simulink model "UAV"  (R2018b)
settings: Solver=FixedStepAuto  StartTime=0.0  StopTime=10.0  RelTol=1e-3  EnableMultiTasking=on
values from neighbouring files (symbols this model uses):
  actuatorCentres = 0.0    [data.sldd]
  datcom : value not decoded    [data.sldd]
  deflectionLimits = -10.0    [data.sldd]
  envConsts = -1.3    [data.sldd]
  vehicle = 5.0    [data.sldd]
undefined symbols (not defined in the file or in its folder): aeroCoeff, Discrete, Time
libraries: simulink x28, ctrlSharedLib x8, arduinolib x7, aerolibasang x6, aerolibactuator x4, aerolibadyn x2, sharedTrackingLibrary x2, aerolibnav x2, shared6dof x1, aerolibanim x1, aerolibatmos2 x1, dspstat3 x1
(part 1 of 3)
settings Model: DataDictionary=data.sldd  VariantConfigurationObject=Sim_Mode  SimulationMode=accelerator  ExtModeTrigDuration=2  Creator=Aliak  LastModifiedBy=Aliak
settings OptimizationCC: DefaultUnderspecifiedDataType=single  EnhancedBackFolding=on  PassReuseOutputArgsAs=Individual arguments  LifeSpan=1  MaxStackSize=64  OptimizeBlockOrder=speed  DifferentSizesBufferReuse=on
settings DebuggingCC: ParameterTunabilityLossMsg=error
settings HardwareCC: ProdBitPerInt=16  ProdBitPerPointer=16  ProdBitPerSizeT=16  ProdBitPerPtrDiffT=16  ProdLargestAtomicFloat=None  ProdWordSize=8  ProdHWDeviceType=Atmel->AVR
settings SFSimCC: MATLABDynamicMemAlloc=off
settings RTWCC: SystemTargetFile=ert.tlc  HardwareBoard=Arduino Uno  TemplateMakefile=ert_default_tmf  GenerateReport=on  Toolchain=Arduino AVR  BuildConfiguration=Faster Runs  IncludeHyperlinkInReport=on  LaunchReport=on  GenerateTraceInfo=on  GenerateTraceReport=on  GenerateTraceReportSl=on  GenerateTraceReportSf=on  GenerateTraceReportEml=on  CheckMdlBeforeBuild=Warning
settings CodeAppCC: ForceParamTrailComments=on  IgnoreCustomStorageClasses=off  OperatorAnnotations=on  SimulinkDataObjDesc=on  SFDataObjDesc=on  InsertBlockDesc=on
settings ERTTargetCC: SupportContinuousTime=on  SupportVariableSizeSignals=on  CastingMode=Standards

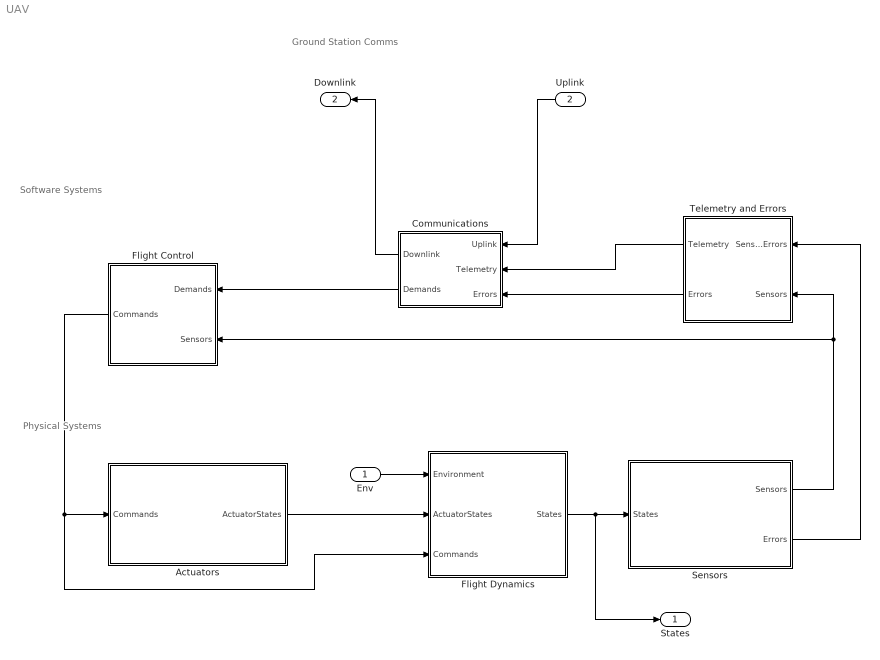
== system UAV ==
  note: Physical Systems
  note: Software Systems
  note: Ground Station Comms
  Env : Inport
  Uplink : Inport  Port=2  OutDataTypeStr=Bus: Uplink
  Actuators : Subsystem  Variant=on
  Communications : Subsystem
  Flight Control : Subsystem
  Flight Dynamics : Subsystem
  Sensors : Subsystem
  Telemetry and Errors : Subsystem  VariantControl=Variant1
  States : Outport  OutDataTypeStr=Bus: States
  Downlink : Outport  Port=2
  wires:
  Flight Dynamics/1(States) -> States/1, Sensors/1(States)
  Sensors/1(Sensors) -> Telemetry and Errors/2(Sensors), Flight Control/2(Sensors)
  Flight Control/1(Commands) -> Actuators/1(Commands), Flight Dynamics/3(Commands)
  Actuators/1(ActuatorStates) -> Flight Dynamics/2(ActuatorStates)
  Env/1 -> Flight Dynamics/1(Environment)
  Communications/2(Demands) -> Flight Control/1(Demands)
  Uplink/1 -> Communications/1(Uplink)
  Communications/1(Downlink) -> Downlink/1
  Sensors/2(Errors) -> Telemetry and Errors/1(SensorErrors)
  Telemetry and Errors/1(Telemetry) -> Communications/2(Telemetry)
  Telemetry and Errors/2(Errors) -> Communications/3(Errors)

== system UAV/Actuators ==
  Commands : Inport
  Model Actuators : Subsystem  VariantControl=SimType == 0
  Real Actuators : Subsystem  VariantControl=SimType == 2
  ActuatorStates : Outport

== system UAV/Communications ==
  Uplink : Inport  OutDataTypeStr=Bus: Uplink
  Telemetry : Inport  Port=2  OutDataTypeStr=Bus: Sensors
  Errors : Inport  Port=3  OutDataTypeStr=Bus: Errors
  Bus Creator : BusCreator  Inputs=6  OutDataTypeStr=Bus: Demands
      settings: InheritFromInputs=off
  Bus Selector : BusSelector  OutputSignals=AutoflightRefValues,ControlOverride
  Bus Selector1 : BusSelector  OutputSignals=FlightMode,HoldAltitude,HoldSpeed,HoldHeading,LLATarget
  Downlink : Outport
  Demands : Outport  Port=2  OutDataTypeStr=Bus: Demands
  wires:
  Uplink/1 -> Bus Selector/1
  Bus Selector/1 -> Bus Selector1/1  "<AutoflightRefValues>"
  Bus Selector1/1 -> Bus Creator/1  "<FlightMode>"
  Bus Selector1/2 -> Bus Creator/2  "<HoldAltitude>"
  Bus Selector1/3 -> Bus Creator/3  "<HoldSpeed>"
  Bus Selector1/4 -> Bus Creator/4  "<HoldHeading>"
  Bus Selector1/5 -> Bus Creator/5  "<LLATarget>"
  Bus Creator/1 -> Demands/1
  Bus Selector/2 -> Bus Creator/6  "<ControlOverride>"

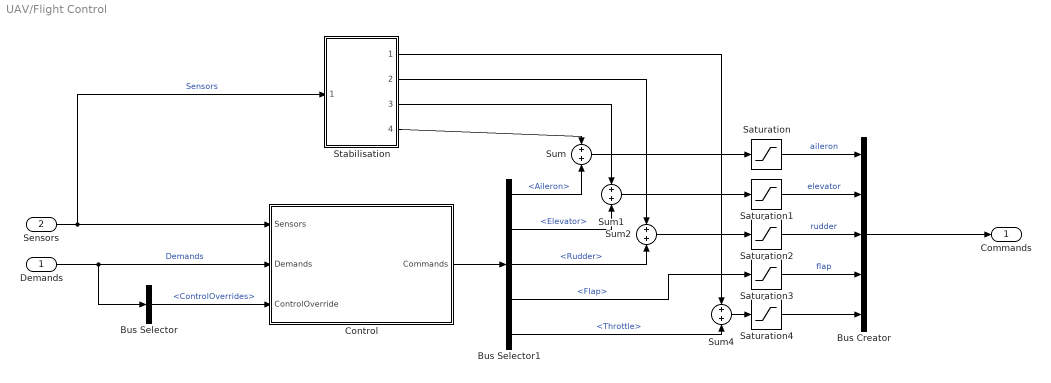
== system UAV/Flight Control ==
  Demands : Inport  OutDataTypeStr=Bus: Demands
  Sensors : Inport  Port=2  OutDataTypeStr=Bus: Sensors
  Bus Creator : BusCreator  Inputs=5  OutDataTypeStr=Bus: Commands
  Bus Selector : BusSelector  OutputSignals=ControlOverrides
  Bus Selector1 : BusSelector  OutputSignals=Aileron,Elevator,Rudder,Flap,Throttle
  Control : Stateflow chart  TreatAsAtomicUnit=on
  Saturation : Saturate  UpperLimit=deflectionLimits.aileron.max  LowerLimit=deflectionLimits.aileron.min
  Saturation1 : Saturate  UpperLimit=deflectionLimits.elevator.max  LowerLimit=deflectionLimits.elevator.min
  Saturation2 : Saturate  UpperLimit=deflectionLimits.rudder.max  LowerLimit=deflectionLimits.rudder.min
  Saturation3 : Saturate  UpperLimit=deflectionLimits.flap.max  LowerLimit=deflectionLimits.flap.min
  Saturation4 : Saturate  UpperLimit=1  LowerLimit=0
  Stabilisation : Subsystem
  Sum{,1..2,4} (4 alike) : Sum
  Commands : Outport
  wires:
  Bus Creator/1 -> Commands/1
  Sum/1 -> Saturation/1
  Sum1/1 -> Saturation1/1
  Sum2/1 -> Saturation2/1
  Saturation/1 -> Bus Creator/1  "aileron"
  Saturation1/1 -> Bus Creator/2  "elevator"
  Saturation2/1 -> Bus Creator/3  "rudder"
  Saturation3/1 -> Bus Creator/4  "flap"
  Control/1(Commands) -> Bus Selector1/1
  Bus Selector1/1 -> Sum/2  "<Aileron>"
  Sensors/1 -> Stabilisation/1(Sensors), Control/1(Sensors)  "Sensors"
  Demands/1 -> Bus Selector/1, Control/2(Demands)  "Demands"
  Bus Selector/1 -> Control/3(ControlOverride)  "<ControlOverrides>"
  Bus Selector1/2 -> Sum1/2  "<Elevator>"
  Bus Selector1/3 -> Sum2/2  "<Rudder>"
  Bus Selector1/4 -> Saturation3/1  "<Flap>"
  Sum4/1 -> Saturation4/1
  Bus Selector1/5 -> Sum4/2  "<Throttle>"
  Saturation4/1 -> Bus Creator/5
  Stabilisation/4(Roll Stab) -> Sum/1
  Stabilisation/3(Pitch Stab) -> Sum1/1
  Stabilisation/2(Yaw Stab) -> Sum2/1
  Stabilisation/1(Stall Stab) -> Sum4/1

== system UAV/Flight Dynamics ==
  Environment : Inport
  ActuatorStates : Inport  Port=2
  Commands : Inport  Port=3  OutDataTypeStr=Bus: Commands
  6DOF EOM : Subsystem  VariantControl=eom3DOF
  Bus Selector : BusSelector  OutputSignals=throttle
  Coeff Model : Subsystem  Commented=on  VariantControl=AeroModel==2
  DATCOM Model : Subsystem  VariantControl=AeroModel==1
  Propulsion : Subsystem
      settings: RTWSystemCode=Inline
  Sum1 : Sum  Inputs=|++  SaturateOnIntegerOverflow=on  InputSameDT=on  OutDataTypeStr=Inherit: Same as first input
  Sum2 : Sum  Inputs=|++  SaturateOnIntegerOverflow=on  InputSameDT=on  OutDataTypeStr=Inherit: Same as first input
  Visualization : Subsystem
  States : Outport  OutDataTypeStr=Bus: States
  wires:
  Commands/1 -> Bus Selector/1
  Sum2/1 -> 6DOF EOM/2(Forces)
  6DOF EOM/1(States) -> DATCOM Model/2(States), States/1, Visualization/1(States)
  Propulsion/1(F) -> Sum2/2
  Propulsion/2(M) -> Sum1/2
  Sum1/1 -> 6DOF EOM/3(Moments)
  Environment/1 -> DATCOM Model/1(Env), 6DOF EOM/1(Env)
  Bus Selector/1 -> Propulsion/1(cmd)  "<throttle>"
  ActuatorStates/1 -> DATCOM Model/3(ActuatorStates)
  DATCOM Model/1(F) -> Sum2/1
  DATCOM Model/2(M) -> Sum1/1

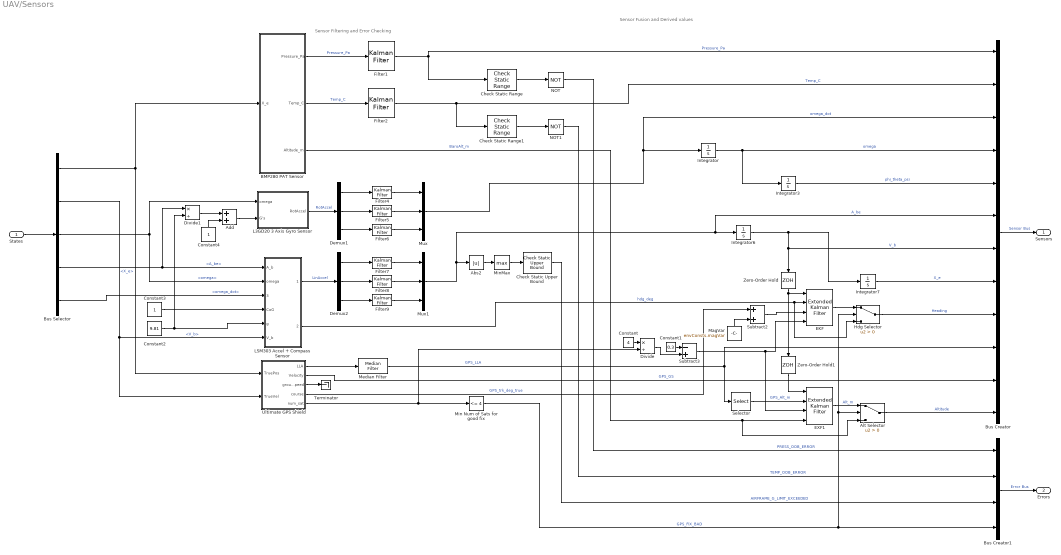
== system UAV/Sensors ==
  note: Sensor Fusion and Derived values
  note: Sensor Filtering and Error Checking
  States : Inport  OutDataTypeStr=Bus: States
  Abs2 : Abs
  Add : Sum
  Alt Selector : Switch  Criteria=u2 > Threshold  OutDataTypeStr=single  SaturateOnIntegerOverflow=on  InputSameDT=on
  "BMP280 PAT Sensor " : Subsystem
  Bus Creator : BusCreator  Inputs=12  OutDataTypeStr=Bus: Sensors
  Bus Creator1 : BusCreator  Inputs=4  OutDataTypeStr=Bus: Errors
  Bus Selector : BusSelector  OutputSignals=X_e,V_b,omega,A_be,omega_dot
  Check Static Range : simulink/Model Verification/Check  Static Range  Description=97025 <= u <= 104325  max=104325  max_included=on  min=97025  min_included=on  enabled=off  stopWhenAssertionFail=off  export=on  icon=graphic
      settings: SourceProductName=Simulink  SourceProductBaseCode=SL
  Check Static Range1 : simulink/Model Verification/Check  Static Range  Description=-10 <= u <= 30  max=30  max_included=on  min=-10  min_included=on  enabled=off  stopWhenAssertionFail=off  export=on  icon=graphic
      settings: SourceProductName=Simulink  SourceProductBaseCode=SL
  Check Static Upper Bound : simulink/Model Verification/Check Static  Upper Bound  Description=u <= 5  max=5  max_included=on  enabled=off  stopWhenAssertionFail=off  export=on  icon=graphic
      settings: SourceProductName=Simulink  SourceProductBaseCode=SL
  Constant : Constant  Value=4
  Constant1 : Constant  Value=0.3
  Constant2 : Constant  Value=9.81
  Constant3 : Constant
  Constant4 : Constant
  Demux1 : Demux  Outputs=3
  Demux2 : Demux  Outputs=3
  Divide : Product  Inputs=*/  OutMin=0.5  OutMax=30  OutDataTypeStr=Inherit: Inherit via back propagation  SaturateOnIntegerOverflow=on
  Divide1 : Product  Inputs=*/
  EKF : sharedTrackingLibrary/Extended Kalman Filter  StateTransitionFcn=headingStateTransitionFunc  HasStateTransitionJacobianFcn=off  HasAdditiveProcessNoise=Additive  ProcessNoise=1  HasTimeVaryingProcessNoise=off  HasStateTransitionFcnExtraArgument=1  InitialState=0  InitialStateCovariance=3  MeasurementFcn1=baroMeasurementFunc  HasMeasurementJacobianFcn1=off  HasMeasurementEnablePort1=off  HasAdditiveMeasurementNoise1=Additive  MeasurementNoise1=0.5  HasTimeVaryingMeasurementNoise1=off  HasMeasurementFcnExtraArgument1=0  MeasurementFcn2=gpsMeasurementFunc  HasMeasurementJacobianFcn2=off  HasMeasurementEnablePort2=off  HasAdditiveMeasurementNoise2=Additive  MeasurementNoise2=1  HasTimeVaryingMeasurementNoise2=on  HasMeasurementFcnExtraArgument2=0  MeasurementFcn3=myMeasurementFcn  HasMeasurementJacobianFcn3=off  HasMeasurementEnablePort3=off  HasAdditiveMeasurementNoise3=Additive  MeasurementNoise3=1  HasTimeVaryingMeasurementNoise3=off  HasMeasurementFcnExtraArgument3=0  MeasurementFcn4=myMeasurementFcn  HasMeasurementJacobianFcn4=off  HasMeasurementEnablePort4=off  HasAdditiveMeasurementNoise4=Additive  MeasurementNoise4=1  HasTimeVaryingMeasurementNoise4=off  HasMeasurementFcnExtraArgument4=0  MeasurementFcn5=myMeasurementFcn  HasMeasurementJacobianFcn5=off  HasMeasurementEnablePort5=off  HasAdditiveMeasurementNoise5=Additive  MeasurementNoise5=1  HasTimeVaryingMeasurementNoise5=off  HasMeasurementFcnExtraArgument5=0  EnableMultirate=off  StateTransitionFcnSampleTime=0.01  MeasurementFcn1SampleTime=0.01  MeasurementFcn2SampleTime=1  MeasurementFcn3SampleTime=1  MeasurementFcn4SampleTime=1  MeasurementFcn5SampleTime=1  UseCurrentEstimator=on  OutputStateCovariance=off  DataType=double  SampleTime=1  NumberOfMeasurements=2
      settings: SourceProductName=Control System Toolbox  SourceProductBaseCode=CT
  EXF1 : sharedTrackingLibrary/Extended Kalman Filter  StateTransitionFcn=altitudeStateTransitionFunc  HasStateTransitionJacobianFcn=off  HasAdditiveProcessNoise=Additive  ProcessNoise=1  HasTimeVaryingProcessNoise=off  HasStateTransitionFcnExtraArgument=1  InitialState=0  InitialStateCovariance=1  MeasurementFcn1=gpsMeasurementFunc  HasMeasurementJacobianFcn1=off  HasMeasurementEnablePort1=off  HasAdditiveMeasurementNoise1=Additive  MeasurementNoise1=1  HasTimeVaryingMeasurementNoise1=on  HasMeasurementFcnExtraArgument1=0  MeasurementFcn2=baroMeasurementFunc  HasMeasurementJacobianFcn2=off  HasMeasurementEnablePort2=off  HasAdditiveMeasurementNoise2=Additive  MeasurementNoise2=0.8  HasTimeVaryingMeasurementNoise2=off  HasMeasurementFcnExtraArgument2=0  MeasurementFcn3=myMeasurementFcn  HasMeasurementJacobianFcn3=off  HasMeasurementEnablePort3=off  HasAdditiveMeasurementNoise3=Additive  MeasurementNoise3=1  HasTimeVaryingMeasurementNoise3=off  HasMeasurementFcnExtraArgument3=0  MeasurementFcn4=myMeasurementFcn  HasMeasurementJacobianFcn4=off  HasMeasurementEnablePort4=off  HasAdditiveMeasurementNoise4=Additive  MeasurementNoise4=1  HasTimeVaryingMeasurementNoise4=off  HasMeasurementFcnExtraArgument4=0  MeasurementFcn5=myMeasurementFcn  HasMeasurementJacobianFcn5=off  HasMeasurementEnablePort5=off  HasAdditiveMeasurementNoise5=Additive  MeasurementNoise5=1  HasTimeVaryingMeasurementNoise5=off  HasMeasurementFcnExtraArgument5=0  EnableMultirate=off  StateTransitionFcnSampleTime=0.01  MeasurementFcn1SampleTime=1  MeasurementFcn2SampleTime=1  MeasurementFcn3SampleTime=1  MeasurementFcn4SampleTime=1  MeasurementFcn5SampleTime=1  UseCurrentEstimator=on  OutputStateCovariance=off  DataType=double  SampleTime=1  NumberOfMeasurements=2
      settings: SourceProductName=Control System Toolbox  SourceProductBaseCode=CT
  Filter1 : ctrlSharedLib/Kalman Filter  TimeDomain=Discrete-Time  UseCurrentEstimator=on  ModelSource=LTI State-Space Variable  ModelSourceVariable=ss(1,[],1,[],1)  A=0.95  B=1  C=1  D=0  NumberOfStates=1  NumberOfInputs=1  NumberOfOutputs=1  InitialEstimateSource=Dialog  X0=101325  P0=10  UseK=off  UseGH=off  NumberOfProcessNoiseInputs=1  G=1  TimeInvariantG=on  H=0  TimeInvariantH=on  Q=0.05  TimeInvariantQ=on  R=1  TimeInvariantR=on  N=0  TimeInvariantN=on  AddInputPort=off  AddEnablePort=off  OutputEstimatedY=off  OutputP=off  Ts=-1
      settings: SourceProductBaseCode=CT
  Filter2 : ctrlSharedLib/Kalman Filter  TimeDomain=Discrete-Time  UseCurrentEstimator=on  ModelSource=LTI State-Space Variable  ModelSourceVariable=ss(1,[],1,[],1)  A=0.95  B=1  C=1  D=0  NumberOfStates=1  NumberOfInputs=1  NumberOfOutputs=1  InitialEstimateSource=Dialog  X0=15  P0=10  UseK=off  UseGH=off  NumberOfProcessNoiseInputs=1  G=1  TimeInvariantG=on  H=0  TimeInvariantH=on  Q=0.05  TimeInvariantQ=on  R=1  TimeInvariantR=on  N=0  TimeInvariantN=on  AddInputPort=off  AddEnablePort=off  OutputEstimatedY=off  OutputP=off  Ts=-1
      settings: SourceProductBaseCode=CT
  Filter4 : ctrlSharedLib/Kalman Filter  TimeDomain=Discrete-Time  UseCurrentEstimator=on  ModelSource=LTI State-Space Variable  ModelSourceVariable=ss(0.95,[],1,[],1/95)  A=0.95  B=1  C=1  D=0  NumberOfStates=1  NumberOfInputs=1  NumberOfOutputs=1  InitialEstimateSource=Dialog  X0=0  P0=10  UseK=off  UseGH=off  NumberOfProcessNoiseInputs=1  G=1  TimeInvariantG=on  H=0  TimeInvariantH=on  Q=0.05  TimeInvariantQ=on  R=0.8  TimeInvariantR=on  N=0  TimeInvariantN=on  AddInputPort=off  AddEnablePort=off  OutputEstimatedY=off  OutputP=off  Ts=-1
      settings: SourceProductBaseCode=CT
  Filter5 : ctrlSharedLib/Kalman Filter  TimeDomain=Discrete-Time  UseCurrentEstimator=on  ModelSource=LTI State-Space Variable  ModelSourceVariable=ss(0.95,[],1,[],1/95)  A=0.95  B=1  C=1  D=0  NumberOfStates=1  NumberOfInputs=1  NumberOfOutputs=1  InitialEstimateSource=Dialog  X0=0  P0=10  UseK=off  UseGH=off  NumberOfProcessNoiseInputs=1  G=1  TimeInvariantG=on  H=0  TimeInvariantH=on  Q=0.05  TimeInvariantQ=on  R=0.8  TimeInvariantR=on  N=0  TimeInvariantN=on  AddInputPort=off  AddEnablePort=off  OutputEstimatedY=off  OutputP=off  Ts=-1
      settings: SourceProductBaseCode=CT
  Filter6 : ctrlSharedLib/Kalman Filter  TimeDomain=Discrete-Time  UseCurrentEstimator=on  ModelSource=LTI State-Space Variable  ModelSourceVariable=ss(0.95,[],1,[],1/95)  A=0.95  B=1  C=1  D=0  NumberOfStates=1  NumberOfInputs=1  NumberOfOutputs=1  InitialEstimateSource=Dialog  X0=0  P0=10  UseK=off  UseGH=off  NumberOfProcessNoiseInputs=1  G=1  TimeInvariantG=on  H=0  TimeInvariantH=on  Q=0.05  TimeInvariantQ=on  R=0.8  TimeInvariantR=on  N=0  TimeInvariantN=on  AddInputPort=off  AddEnablePort=off  OutputEstimatedY=off  OutputP=off  Ts=-1
      settings: SourceProductBaseCode=CT
  Filter7 : ctrlSharedLib/Kalman Filter  TimeDomain=Discrete-Time  UseCurrentEstimator=on  ModelSource=LTI State-Space Variable  ModelSourceVariable=ss(0.95,[],1,[],1/100)  A=0.95  B=1  C=1  D=0  NumberOfStates=1  NumberOfInputs=1  NumberOfOutputs=1  InitialEstimateSource=Dialog  X0=0  P0=10  UseK=off  UseGH=off  NumberOfProcessNoiseInputs=1  G=1  TimeInvariantG=on  H=0  TimeInvariantH=on  Q=0.05  TimeInvariantQ=on  R=1  TimeInvariantR=on  N=0  TimeInvariantN=on  AddInputPort=off  AddEnablePort=off  OutputEstimatedY=off  OutputP=off  Ts=-1
      settings: SourceProductBaseCode=CT
  Filter8 : ctrlSharedLib/Kalman Filter  TimeDomain=Discrete-Time  UseCurrentEstimator=on  ModelSource=LTI State-Space Variable  ModelSourceVariable=ss(0.95,[],1,[],1/100)  A=0.95  B=1  C=1  D=0  NumberOfStates=1  NumberOfInputs=1  NumberOfOutputs=1  InitialEstimateSource=Dialog  X0=0  P0=10  UseK=off  UseGH=off  NumberOfProcessNoiseInputs=1  G=1  TimeInvariantG=on  H=0  TimeInvariantH=on  Q=0.05  TimeInvariantQ=on  R=1  TimeInvariantR=on  N=0  TimeInvariantN=on  AddInputPort=off  AddEnablePort=off  OutputEstimatedY=off  OutputP=off  Ts=-1
      settings: SourceProductBaseCode=CT
  Filter9 : ctrlSharedLib/Kalman Filter  TimeDomain=Discrete-Time  UseCurrentEstimator=on  ModelSource=LTI State-Space Variable  ModelSourceVariable=ss(0.95,[],1,[],1/100)  A=0.95  B=1  C=1  D=0  NumberOfStates=1  NumberOfInputs=1  NumberOfOutputs=1  InitialEstimateSource=Dialog  X0=0  P0=10  UseK=off  UseGH=off  NumberOfProcessNoiseInputs=1  G=1  TimeInvariantG=on  H=0  TimeInvariantH=on  Q=0.05  TimeInvariantQ=on  R=1  TimeInvariantR=on  N=0  TimeInvariantN=on  AddInputPort=off  AddEnablePort=off  OutputEstimatedY=off  OutputP=off  Ts=-1
      settings: SourceProductBaseCode=CT
  Hdg Selector : Switch  Criteria=u2 > Threshold  OutDataTypeStr=Inherit: Inherit via back propagation  SaturateOnIntegerOverflow=on  InputSameDT=on
  Integrator{,3,6..7} (4 alike) : Integrator
  L3GD20 3 Axis Gyro Sensor : Subsystem
  LSM303 Accel + Compass Sensor : Subsystem
  MagVar : Constant  Value=envConsts.magVar
  Median Filter : dspstat3/Median Filter  WindowLength=20  SimulateUsing=Code generation
      settings: SourceProductName=DSP System Toolbox  SourceProductBaseCode=DS
  Min Num of Sats for good fix : simulink/Logic and Bit Operations/Compare To Constant  relop=<=  const=4  OutDataTypeStr=boolean
  MinMax : MinMax  Function=max
  Mux : Mux  Inputs=3
  Mux1 : Mux  Inputs=3
  NOT : Logic  Operator=NOT  IconShape=distinctive  AllPortsSameDT=off  OutDataTypeStr=boolean
  NOT1 : Logic  Operator=NOT  IconShape=distinctive  AllPortsSameDT=off  OutDataTypeStr=boolean
  Selector : Selector  InputPortWidth=3  IndexOptions=Index vector (dialog)  Indices=[3]  OutputSizes=1
  Subtract2 : Sum
  Subtract3 : Sum  Inputs=-+
  Terminator : Terminator
  Ultimate GPS Shield : Subsystem
  Zero-Order Hold : ZeroOrderHold  SampleTime=1/100
  Zero-Order Hold1 : ZeroOrderHold
  Sensors : Outport
  Errors : Outport  Port=2
  wires:
  Bus Selector/4 -> Divide1/1, LSM303 Accel + Compass Sensor/1(A_b)  "<A_be>"
  Constant4/1 -> Add/2
  Add/1 -> L3GD20 3 Axis Gyro Sensor/2(G's)
  Divide1/1 -> Add/1
  Bus Selector/5 -> LSM303 Accel + Compass Sensor/3(omega_dot)  "<omega_dot>"
  Bus Selector/2 -> Ultimate GPS Shield/2(TrueVel), LSM303 Accel + Compass Sensor/6(V_b)  "<V_b>"
  Constant1/1 -> Subtract3/1
  Integrator/1 -> Integrator3/1, Bus Creator/4  "omega"
  Demux1/3 -> Filter6/1
  "BMP280 PAT Sensor "/1(Pressure_Pa) -> Filter1/1  "Pressure_Pa"
  Bus Selector/1 -> Ultimate GPS Shield/1(TruePos), "BMP280 PAT Sensor "/1(X_e)  "<X_e>"
  Bus Selector/3 -> L3GD20 3 Axis Gyro Sensor/1(omega), LSM303 Accel + Compass Sensor/2(omega)  "<omega>"
  Constant3/1 -> LSM303 Accel + Compass Sensor/4(CoG)
  Demux1/2 -> Filter5/1
  Constant2/1 -> LSM303 Accel + Compass Sensor/5(g), Divide1/2
  Integrator3/1 -> Bus Creator/5  "phi_theta_psi"
  Mux/1 -> Integrator/1, Bus Creator/3  "omega_dot"
  EXF1/1 -> Alt Selector/1  "Alt_m"
  Min Num of Sats for good fix/1 -> Bus Creator1/4, Alt Selector/2, Hdg Selector/2  "GPS_FIX_BAD"
  Subtract3/1 -> EXF1/3, EKF/4
  Divide/1 -> Subtract3/2
  EKF/1 -> Hdg Selector/1
  Constant/1 -> Divide/1
  Selector/1 -> EXF1/2  "GPS_Alt_m"
  Demux2/1 -> Filter7/1
  Filter1/1 -> Check Static Range/1, Bus Creator/1  "Pressure_Pa"
  Zero-Order Hold/1 -> Zero-Order Hold1/1, EKF/1
  Integrator6/1 -> Integrator7/1, Bus Creator/7, Zero-Order Hold/1  "V_b"
  Check Static Range/1 -> NOT/1
  Alt Selector/1 -> Bus Creator/12  "Altitude"
  NOT1/1 -> Bus Creator1/2  "TEMP_OOB_ERROR"
  Filter4/1 -> Mux/1
  Hdg Selector/1 -> Bus Creator/9  "Heading"
  Ultimate GPS Shield/1(LLA) -> Median Filter/1
  Subtract2/1 -> EKF/3
  Ultimate GPS Shield/5(num_sat) -> Divide/2, Min Num of Sats for good fix/1
  Demux1/1 -> Filter4/1
  Filter9/1 -> Mux1/3
  Demux2/3 -> Filter9/1
  Demux2/2 -> Filter8/1
  Median Filter/1 -> Selector/1, Bus Creator/10  "GPS_LLA"
  Filter6/1 -> Mux/3
  LSM303 Accel + Compass Sensor/1(LinAccel) -> Demux2/1  "LinAccel"
  "BMP280 PAT Sensor "/3(Altitude_m) -> EXF1/4, Alt Selector/3  "BaroAlt_m"
  Filter8/1 -> Mux1/2
  Abs2/1 -> MinMax/1
  Filter5/1 -> Mux/2
  MinMax/1 -> Check Static Upper Bound/1
  Filter2/1 -> Bus Creator/2, Check Static Range1/1  "Temp_C"
  Integrator7/1 -> Bus Creator/8  "X_e"
  Check Static Upper Bound/1 -> Bus Creator1/3  "AIRFRAME_G_LIMIT_EXCEEDED"
  MagVar/1 -> Subtract2/2
  Filter7/1 -> Mux1/1
  "BMP280 PAT Sensor "/2(Temp_C) -> Filter2/1  "Temp_C"
  Mux1/1 -> Integrator6/1, Bus Creator/6, Abs2/1  "A_be"
  L3GD20 3 Axis Gyro Sensor/1(RotAccel) -> Demux1/1  "RotAccel"
  LSM303 Accel + Compass Sensor/2(hdg_deg) -> EKF/2, Hdg Selector/3  "hdg_deg"
  Ultimate GPS Shield/3(groundspeed) -> Terminator/1
  Check Static Range1/1 -> NOT1/1
  Ultimate GPS Shield/4(course) -> Subtract2/1  "GPS_trk_deg_true"
  Ultimate GPS Shield/2(Velocity) -> Bus Creator/11  "GPS_GS"
  States/1 -> Bus Selector/1
  Zero-Order Hold1/1 -> EXF1/1
  NOT/1 -> Bus Creator1/1  "PRESS_OOB_ERROR"
  Bus Creator/1 -> Sensors/1  "Sensor Bus"
  Bus Creator1/1 -> Errors/1  "Error Bus"

== system UAV/Telemetry and Errors ==
  SensorErrors : Inport
  Sensors : Inport  Port=2
  Altitude : Scope
  Body Angles : Scope  NumInputPorts=3
  Body Velocities : Scope  NumInputPorts=3
  Bus Selector : BusSelector  OutputSignals=phi_theta_psi,V_b,Altitude,Heading
  Demux : Demux  Outputs=3
  Demux1 : Demux  Outputs=3
  Heading : Scope
  Telemetry : Outport
  Errors : Outport  Port=2
  wires:
  Sensors/1 -> Bus Selector/1, Telemetry/1
  SensorErrors/1 -> Errors/1
  Bus Selector/1 -> Demux/1  "<phi_theta_psi>"
  Demux/1 -> Body Angles/1  "Roll Angle"
  Demux/2 -> Body Angles/2  "Pitch Angle"
  Demux/3 -> Body Angles/3  "Yaw Angle"
  Bus Selector/2 -> Demux1/1  "<V_b>"
  Demux1/1 -> Body Velocities/1  "X Vel"
  Demux1/2 -> Body Velocities/2  "Y Vel"
  Demux1/3 -> Body Velocities/3  "Z Vel"
  Bus Selector/3 -> Altitude/1  "<Altitude>"
  Bus Selector/4 -> Heading/1  "<Heading>"

== system UAV/Actuators/Model Actuators ==
  Commands : Inport
  Bus Creator : BusCreator  Inputs=4  OutDataTypeStr=Bus: ActuatorStates
  Bus Selector : BusSelector  OutputSignals=AileronCmd,ElevatorCmd,RudderCmd,FlapCmd
  Linear Second-Order Actuator{,1..3} (4 alike) : aerolibactuator/Linear Second-Order Actuator  wn_fin=1  z_fin=0.3  fin_act_0=0  fin_act_vel=0
      settings: SourceProductName=Aerospace Blockset  SourceProductBaseCode=AE
  Saturation : Saturate  UpperLimit=deflectionLimits.aileron.max  LowerLimit=deflectionLimits.aileron.min
  Saturation1 : Saturate  UpperLimit=deflectionLimits.elevator.max  LowerLimit=deflectionLimits.elevator.min
  Saturation2 : Saturate  UpperLimit=deflectionLimits.rudder.max  LowerLimit=deflectionLimits.rudder.min
  Saturation3 : Saturate  UpperLimit=deflectionLimits.flap.max  LowerLimit=deflectionLimits.flap.min
  ActuatorStates : Outport
  wires:
  Bus Selector/3 -> Saturation2/1  "<RudderCmd>"
  Commands/1 -> Bus Selector/1
  Bus Selector/4 -> Saturation3/1  "<FlapCmd>"
  Bus Selector/1 -> Saturation/1  "<AileronCmd>"
  Bus Selector/2 -> Saturation1/1  "<ElevatorCmd>"
  Saturation/1 -> Linear Second-Order Actuator/1
  Saturation1/1 -> Linear Second-Order Actuator1/1
  Saturation2/1 -> Linear Second-Order Actuator2/1
  Saturation3/1 -> Linear Second-Order Actuator3/1
  Linear Second-Order Actuator1/1 -> Bus Creator/2  "Elevator"
  Linear Second-Order Actuator/1 -> Bus Creator/1  "Aileron"
  Linear Second-Order Actuator2/1 -> Bus Creator/3  "Rudder"
  Linear Second-Order Actuator3/1 -> Bus Creator/4  "Flap"
  Bus Creator/1 -> ActuatorStates/1

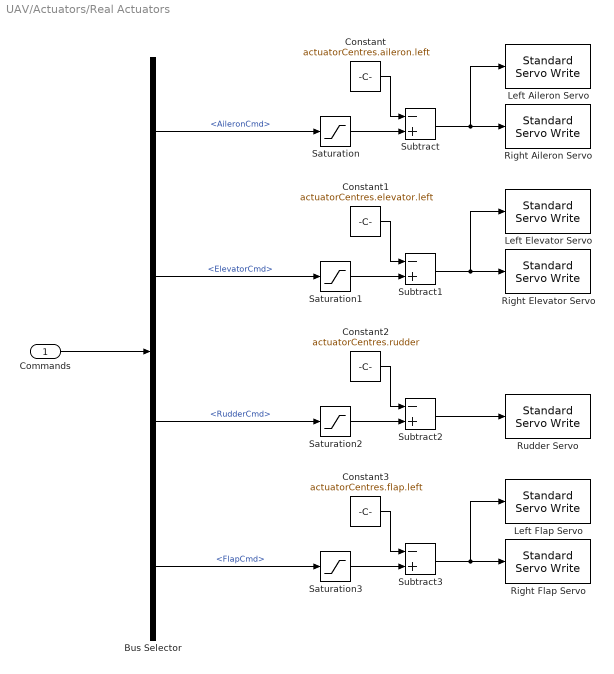
== system UAV/Actuators/Real Actuators ==
  Commands : Inport
  Bus Selector : BusSelector  OutputSignals=AileronCmd,ElevatorCmd,RudderCmd,FlapCmd
  Constant : Constant  Value=actuatorCentres.aileron.left
  Constant1 : Constant  Value=actuatorCentres.elevator.left
  Constant2 : Constant  Value=actuatorCentres.rudder
  Constant3 : Constant  Value=actuatorCentres.flap.left
  Left Aileron Servo : arduinolib/Standard Servo Write  pinNumber=servoPins.aileron.left  ServoIndex=0  blockPlatform=ARDUINO
      settings: SourceProductName=Simulink Support Package for Arduino Hardware
  Left Elevator Servo : arduinolib/Standard Servo Write  pinNumber=servoPins.elevator.left  ServoIndex=0  blockPlatform=ARDUINO
      settings: SourceProductName=Simulink Support Package for Arduino Hardware
  Left Flap Servo : arduinolib/Standard Servo Write  pinNumber=servoPins.flap.left  ServoIndex=0  blockPlatform=ARDUINO
      settings: SourceProductName=Simulink Support Package for Arduino Hardware
  Right Aileron Servo : arduinolib/Standard Servo Write  pinNumber=servoPins.aileron.right  ServoIndex=0  blockPlatform=ARDUINO
      settings: SourceProductName=Simulink Support Package for Arduino Hardware
  Right Elevator Servo : arduinolib/Standard Servo Write  pinNumber=servoPins.elevator.right  ServoIndex=0  blockPlatform=ARDUINO
      settings: SourceProductName=Simulink Support Package for Arduino Hardware
  Right Flap Servo : arduinolib/Standard Servo Write  pinNumber=servoPins.flap.right  ServoIndex=0  blockPlatform=ARDUINO
      settings: SourceProductName=Simulink Support Package for Arduino Hardware
  Rudder Servo : arduinolib/Standard Servo Write  pinNumber=servoPins.rudder  ServoIndex=0  blockPlatform=ARDUINO
      settings: SourceProductName=Simulink Support Package for Arduino Hardware
  Saturation : Saturate  UpperLimit=deflectionLimits.aileron.max  LowerLimit=deflectionLimits.aileron.min
  Saturation1 : Saturate  UpperLimit=deflectionLimits.elevator.max  LowerLimit=deflectionLimits.elevator.min
  Saturation2 : Saturate  UpperLimit=deflectionLimits.rudder.max  LowerLimit=deflectionLimits.rudder.min
  Saturation3 : Saturate  UpperLimit=deflectionLimits.flap.max  LowerLimit=deflectionLimits.flap.min
  Subtract{,1..3} (4 alike) : Sum  Inputs=-+
  wires:
  Saturation/1 -> Subtract/2
  Bus Selector/3 -> Saturation2/1  "<RudderCmd>"
  Commands/1 -> Bus Selector/1
  Bus Selector/4 -> Saturation3/1  "<FlapCmd>"
  Subtract3/1 -> Right Flap Servo/1, Left Flap Servo/1
  Bus Selector/1 -> Saturation/1  "<AileronCmd>"
  Constant2/1 -> Subtract2/1
  Subtract2/1 -> Rudder Servo/1
  Saturation3/1 -> Subtract3/2
  Saturation2/1 -> Subtract2/2
  Saturation1/1 -> Subtract1/2
  Bus Selector/2 -> Saturation1/1  "<ElevatorCmd>"
  Subtract/1 -> Right Aileron Servo/1, Left Aileron Servo/1
  Subtract1/1 -> Right Elevator Servo/1, Left Elevator Servo/1
  Constant/1 -> Subtract/1
  Constant1/1 -> Subtract1/1
  Constant3/1 -> Subtract3/1

== system UAV/Flight Control/Control/Guidance.Altitude.ALT ==
  Sensors : Inport  OutDataTypeStr=Bus: Sensors
  Demands : Inport  Port=2  OutDataTypeStr=Bus: Demands
  Action Port : ActionPort
      settings: CopyFcn=Stateflow.SLINSF.SimulinkMan.removeBlockPreDeleteFcn  PreDeleteFcn=Stateflow.SLINSF.SimulinkMan.unsafePredeleteFcn
  Altitude Hold : Subsystem
  Bus Creator : BusCreator  Inputs=1
  Bus Selector : BusSelector  OutputSignals=Altitude,euler_angles
  Bus Selector1 : BusSelector  OutputSignals=Altitude
  Rate Limiter : RateLimiter  SampleTimeMode=inherited
  Selector2 : Selector  InputPortWidth=3  IndexOptions=Index vector (dialog)  Indices=[2]  OutputSizes=1
  Commands : Outport
  wires:
  Bus Creator/1 -> Commands/1
  Altitude Hold/1(Elevator) -> Bus Creator/1
  Selector2/1 -> Altitude Hold/3(theta)
  Sensors/1 -> Bus Selector/1
  Demands/1 -> Bus Selector1/1
  Bus Selector/1 -> Altitude Hold/1(ALT)  "<Altitude>"
  Bus Selector/2 -> Selector2/1  "<euler_angles>"
  Bus Selector1/1 -> Rate Limiter/1  "<Altitude>"
  Rate Limiter/1 -> Altitude Hold/2(Demanded ALT)

== system UAV/Flight Control/Control/Guidance.Autoclimb ==
  Action Port : ActionPort
      settings: CopyFcn=Stateflow.SLINSF.SimulinkMan.removeBlockPreDeleteFcn  PreDeleteFcn=Stateflow.SLINSF.SimulinkMan.unsafePredeleteFcn
  Constant : Constant
  Mux : Mux
  Commands : Outport
  wires:
  Mux/1 -> Commands/1
  Constant/1 -> Mux/4

== system UAV/Flight Control/Control/Guidance.Heading.HDG_ALT ==
  Sensors : Inport  OutDataTypeStr=Bus: Sensors
  Demands : Inport  Port=2  OutDataTypeStr=Bus: Demands
  Action Port : ActionPort
      settings: CopyFcn=Stateflow.SLINSF.SimulinkMan.removeBlockPreDeleteFcn  PreDeleteFcn=Stateflow.SLINSF.SimulinkMan.unsafePredeleteFcn
  Altitude Hold : Subsystem
      settings: UndoDeleteFcn=Stateflow.SLINSF.SimulinkMan.restorePreDeleteFcn  PreDeleteFcn=Stateflow.SLINSF.SimulinkMan.removePreDeleteFcn
  Bus Creator : BusCreator  Inputs=2
  Bus Selector : BusSelector  OutputSignals=Heading,euler_angles,Altitude
  Bus Selector1 : BusSelector  OutputSignals=Heading,Altitude
  Heading Hold : Subsystem
  Rate Limiter : RateLimiter  SampleTimeMode=inherited
  Rate Limiter1 : RateLimiter  SampleTimeMode=inherited
  Selector : Selector  InputPortWidth=3  IndexOptions=Index vector (dialog)  Indices=[1]  OutputSizes=1
  Selector2 : Selector  InputPortWidth=3  IndexOptions=Index vector (dialog)  Indices=[2]  OutputSizes=1
  Commands : Outport
  wires:
  Heading Hold/1(Aileron) -> Bus Creator/1  "Aileron"
  Bus Creator/1 -> Commands/1
  Altitude Hold/1(Elevator) -> Bus Creator/2  "Elevator"
  Selector2/1 -> Altitude Hold/3(theta)
  Sensors/1 -> Bus Selector/1
  Selector/1 -> Heading Hold/3(Current Roll Angle)
  Demands/1 -> Bus Selector1/1
  Bus Selector/3 -> Altitude Hold/1(ALT)  "<Altitude>"
  Bus Selector1/1 -> Rate Limiter/1  "<Heading>"
  Bus Selector/1 -> Heading Hold/1(Current Heading)  "<Heading>"
  Bus Selector/2 -> Selector2/1, Selector/1  "<euler_angles>"
  Bus Selector1/2 -> Rate Limiter1/1  "<Altitude>"
  Rate Limiter/1 -> Heading Hold/2(Demanded Heading)
  Rate Limiter1/1 -> Altitude Hold/2(ALT Demand)

== system UAV/Flight Control/Control/Guidance.Heading1.HDG ==
  Sensors : Inport  OutDataTypeStr=Bus: Sensors
  Demands : Inport  Port=2  OutDataTypeStr=Bus: Demands
  Action Port : ActionPort
      settings: CopyFcn=Stateflow.SLINSF.SimulinkMan.removeBlockPreDeleteFcn  PreDeleteFcn=Stateflow.SLINSF.SimulinkMan.unsafePredeleteFcn
  Bus Creator : BusCreator  Inputs=1
  Bus Selector : BusSelector  OutputSignals=Heading,euler_angles
  Bus Selector1 : BusSelector  OutputSignals=Heading
  Heading Hold : Subsystem
  Rate Limiter : RateLimiter  SampleTimeMode=inherited
  Selector : Selector  InputPortWidth=3  IndexOptions=Index vector (dialog)  Indices=[1]  OutputSizes=1
  Command : Outport  OutDataTypeStr=Bus: Commands
  wires:
  Bus Creator/1 -> Command/1
  Heading Hold/1(Aileron Command) -> Bus Creator/1  "Aileron"
  Sensors/1 -> Bus Selector/1
  Selector/1 -> Heading Hold/3(Current Roll Angle)
  Demands/1 -> Bus Selector1/1
  Bus Selector1/1 -> Rate Limiter/1  "<Heading>"
  Bus Selector/1 -> Heading Hold/1(Current Heading)  "<Heading>"
  Bus Selector/2 -> Selector/1  "<euler_angles>"
  Rate Limiter/1 -> Heading Hold/2(Demanded Heading)

== system UAV/Flight Control/Control/Guidance.Manual ==
  Control Overrides : Inport  OutDataTypeStr=Bus: ControlOverrides
  Action Port : ActionPort
      settings: CopyFcn=Stateflow.SLINSF.SimulinkMan.removeBlockPreDeleteFcn  PreDeleteFcn=Stateflow.SLINSF.SimulinkMan.unsafePredeleteFcn
  Bus Creator : BusCreator  Inputs=5
  Bus Selector : BusSelector  OutputSignals=Aileron,Elevator,Rudder,Flap,Throttle
  Rate Limiter{,1..4} (5 alike) : RateLimiter  SampleTimeMode=inherited
  Commands : Outport
  wires:
  Control Overrides/1 -> Bus Selector/1
  Bus Creator/1 -> Commands/1
  Bus Selector/1 -> Rate Limiter3/1  "<Aileron>"
  Bus Selector/2 -> Rate Limiter2/1  "<Elevator>"
  Bus Selector/3 -> Rate Limiter1/1  "<Rudder>"
  Bus Selector/5 -> Rate Limiter4/1  "<Throttle>"
  Bus Selector/4 -> Rate Limiter/1  "<Flap>"
  Rate Limiter/1 -> Bus Creator/4
  Rate Limiter3/1 -> Bus Creator/1
  Rate Limiter2/1 -> Bus Creator/2
  Rate Limiter1/1 -> Bus Creator/3
  Rate Limiter4/1 -> Bus Creator/5

== system UAV/Flight Control/Control/Guidance.Speed.SPD_HDG_ALT ==
  Sensors : Inport  OutDataTypeStr=Bus: Sensors
  Demands : Inport  Port=2  OutDataTypeStr=Bus: Demands
  Action Port : ActionPort
      settings: CopyFcn=Stateflow.SLINSF.SimulinkMan.removeBlockPreDeleteFcn  PreDeleteFcn=Stateflow.SLINSF.SimulinkMan.unsafePredeleteFcn
  Altitude Hold : Subsystem
  Bus Creator : BusCreator  Inputs=3
  Bus Selector : BusSelector  OutputSignals=Heading,euler_angles,Altitude,V_b
  Bus Selector1 : BusSelector  OutputSignals=Heading,Altitude,GroundSpeed
  Heading Hold : Subsystem
  Rate Limiter : RateLimiter  SampleTimeMode=inherited
  Rate Limiter1 : RateLimiter  SampleTimeMode=inherited
  Rate Limiter2 : RateLimiter  SampleTimeMode=inherited
  Selector : Selector  InputPortWidth=3  IndexOptions=Index vector (dialog)  Indices=[1]  OutputSizes=1
  Selector1 : Selector  InputPortWidth=3  IndexOptions=Index vector (dialog)  Indices=[1]  OutputSizes=1
  Selector2 : Selector  InputPortWidth=3  IndexOptions=Index vector (dialog)  Indices=[2]  OutputSizes=1
  Speed Hold : Subsystem
  Commands : Outport
  wires:
  Heading Hold/1(Aileron) -> Bus Creator/1  "Aileron"
  Bus Creator/1 -> Commands/1
  Speed Hold/1(Throttle) -> Bus Creator/3  "Throttle"
  Altitude Hold/1(Elevator) -> Bus Creator/2  "Elevator"
  Bus Selector/1 -> Heading Hold/1(Current Heading)  "<Heading>"
  Bus Selector/4 -> Selector1/1  "<V_b>"
  Sensors/1 -> Bus Selector/1
  Demands/1 -> Bus Selector1/1
  Selector/1 -> Heading Hold/3(Current Roll Angle)
  Bus Selector/2 -> Selector2/1, Selector/1  "<euler_angles>"
  Bus Selector1/1 -> Rate Limiter/1  "<Heading>"
  Bus Selector1/3 -> Rate Limiter2/1  "<GroundSpeed>"
  Selector1/1 -> Speed Hold/1(V)
  Selector2/1 -> Altitude Hold/3(theta)
  Bus Selector1/2 -> Rate Limiter1/1  "<Altitude>"
  Bus Selector/3 -> Altitude Hold/1(Altitude)  "<Altitude>"
  Rate Limiter/1 -> Heading Hold/2(Demanded Heading)
  Rate Limiter1/1 -> Altitude Hold/2(Demanded Altitude)
  Rate Limiter2/1 -> Speed Hold/2(Demanded V)

== system UAV/Flight Control/Control/Guidance.Speed1.SPD_HDG ==
  Sensors : Inport  OutDataTypeStr=Bus: Sensors
  Demands : Inport  Port=2  OutDataTypeStr=Bus: Demands
  Action Port : ActionPort
      settings: CopyFcn=Stateflow.SLINSF.SimulinkMan.removeBlockPreDeleteFcn  PreDeleteFcn=Stateflow.SLINSF.SimulinkMan.unsafePredeleteFcn
  Bus Creator : BusCreator  Inputs=2
  Bus Selector : BusSelector  OutputSignals=Heading,euler_angles,V_b
  Bus Selector1 : BusSelector  OutputSignals=Heading,GroundSpeed
  Heading Hold : Subsystem
  Rate Limiter : RateLimiter  SampleTimeMode=inherited
  Rate Limiter1 : RateLimiter  SampleTimeMode=inherited
  Selector : Selector  InputPortWidth=3  IndexOptions=Index vector (dialog)  Indices=[1]  OutputSizes=1
  Selector1 : Selector  InputPortWidth=3  IndexOptions=Index vector (dialog)  Indices=[1]  OutputSizes=1
  Speed Hold : Subsystem
  Commands : Outport
  wires:
  Bus Creator/1 -> Commands/1
  Heading Hold/1(Aileron) -> Bus Creator/1  "Aileron"
  Speed Hold/1(Throttle) -> Bus Creator/2  "Throttle"
  Sensors/1 -> Bus Selector/1
  Bus Selector/1 -> Heading Hold/1(Current Heading)  "<Heading>"
  Demands/1 -> Bus Selector1/1
  Bus Selector1/1 -> Rate Limiter/1  "<Heading>"
  Bus Selector1/2 -> Rate Limiter1/1  "<GroundSpeed>"
  Bus Selector/2 -> Selector/1  "<euler_angles>"
  Bus Selector/3 -> Selector1/1  "<V_b>"
  Selector/1 -> Heading Hold/3(Current Roll Angle)
  Selector1/1 -> Speed Hold/1(V)
  Rate Limiter/1 -> Heading Hold/2(Demanded Heading)
  Rate Limiter1/1 -> Speed Hold/2(V Demand)

== system UAV/Flight Control/Control/Guidance.Speed2.SPD_ALT ==
  Sensors : Inport  OutDataTypeStr=Bus: Sensors
  Demands : Inport  Port=2  OutDataTypeStr=Bus: Demands
  Action Port : ActionPort
      settings: CopyFcn=Stateflow.SLINSF.SimulinkMan.removeBlockPreDeleteFcn  PreDeleteFcn=Stateflow.SLINSF.SimulinkMan.unsafePredeleteFcn
  Altitude Hold : Subsystem
      settings: UndoDeleteFcn=Stateflow.SLINSF.SimulinkMan.restorePreDeleteFcn  PreDeleteFcn=Stateflow.SLINSF.SimulinkMan.removePreDeleteFcn
  Bus Creator : BusCreator  Inputs=2
  Bus Selector : BusSelector  OutputSignals=V_b,Altitude,euler_angles
  Bus Selector1 : BusSelector  OutputSignals=Heading,Altitude,GroundSpeed
  Rate Limiter : RateLimiter  SampleTimeMode=inherited
  Rate Limiter1 : RateLimiter  SampleTimeMode=inherited
  Selector1 : Selector  InputPortWidth=3  IndexOptions=Index vector (dialog)  Indices=[1]  OutputSizes=1
  Selector2 : Selector  InputPortWidth=3  IndexOptions=Index vector (dialog)  Indices=[2]  OutputSizes=1
  Speed Hold : Subsystem
      settings: UndoDeleteFcn=Stateflow.SLINSF.SimulinkMan.restorePreDeleteFcn  PreDeleteFcn=Stateflow.SLINSF.SimulinkMan.removePreDeleteFcn
  Commands : Outport
  wires:
  Bus Creator/1 -> Commands/1
  Speed Hold/1(Throttle) -> Bus Creator/1  "Throttle"
  Altitude Hold/1(Elevator) -> Bus Creator/2  "Elevator"
  Selector2/1 -> Altitude Hold/3(theta)
  Sensors/1 -> Bus Selector/1
  Bus Selector/1 -> Selector1/1  "<V_b>"
  Bus Selector1/3 -> Rate Limiter/1  "<GroundSpeed>"
  Selector1/1 -> Speed Hold/1(V)
  Demands/1 -> Bus Selector1/1
  Bus Selector/2 -> Altitude Hold/1(ALT)  "<Altitude>"
  Bus Selector/3 -> Selector2/1  "<euler_angles>"
  Bus Selector1/2 -> Rate Limiter1/1  "<Altitude>"
  Rate Limiter/1 -> Speed Hold/2(V Demand)
  Rate Limiter1/1 -> Altitude Hold/2(ALT Demand)

== system UAV/Flight Control/Control/Guidance.Speed3.SPD ==
  Sensors : Inport  OutDataTypeStr=Bus: Sensors
  Demands : Inport  Port=2  OutDataTypeStr=Bus: Demands
  Action Port : ActionPort
      settings: CopyFcn=Stateflow.SLINSF.SimulinkMan.removeBlockPreDeleteFcn  PreDeleteFcn=Stateflow.SLINSF.SimulinkMan.unsafePredeleteFcn
  Bus Creator : BusCreator  Inputs=1
  Bus Selector : BusSelector  OutputSignals=V_b
  Bus Selector1 : BusSelector  OutputSignals=GroundSpeed
  Rate Limiter : RateLimiter  SampleTimeMode=inherited
  Selector1 : Selector  InputPortWidth=3  IndexOptions=Index vector (dialog)  Indices=[1]  OutputSizes=1
  Speed Hold : Subsystem
  Commands : Outport
  wires:
  Bus Creator/1 -> Commands/1
  Speed Hold/1(Throttle) -> Bus Creator/1
  Sensors/1 -> Bus Selector/1
  Bus Selector/1 -> Selector1/1  "<V_b>"
  Selector1/1 -> Speed Hold/1(V)
  Demands/1 -> Bus Selector1/1
  Bus Selector1/1 -> Rate Limiter/1  "<GroundSpeed>"
  Rate Limiter/1 -> Speed Hold/2(Demanded V)

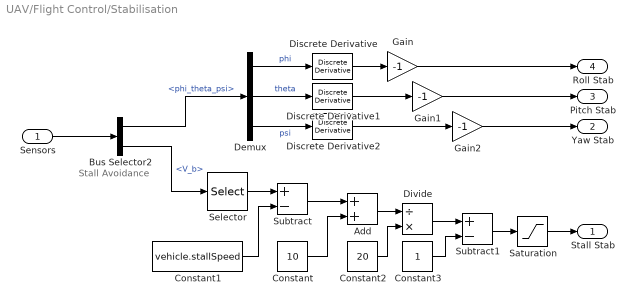
== system UAV/Flight Control/Stabilisation ==
  note: Stall Avoidance
  Sensors : Inport
  Add : Sum
  Bus Selector2 : BusSelector  OutputSignals=phi_theta_psi,V_b
  Constant : Constant  Value=10
  Constant1 : Constant  Value=vehicle.stallSpeed
  Constant2 : Constant  Value=20
  Constant3 : Constant
  Demux : Demux  Outputs=3
  Discrete Derivative : simulink/Discrete/Discrete Derivative  gainval=1.0  ICPrevScaledInput=0.0  OutMin=[]  OutMax=[]  OutDataType=fixdt(1, 16)  OutScaling=2^-10  DoSatur=off
  Discrete Derivative1 : simulink/Discrete/Discrete Derivative  gainval=1.0  ICPrevScaledInput=0.0  OutMin=[]  OutMax=[]  OutDataType=fixdt(1, 16)  OutScaling=2^-10  DoSatur=off
  Discrete Derivative2 : simulink/Discrete/Discrete Derivative  gainval=1.0  ICPrevScaledInput=0.0  OutMin=[]  OutMax=[]  OutDataType=fixdt(1, 16)  OutScaling=2^-10  DoSatur=off
  Divide : Product  Inputs=/*
  Gain : Gain  Gain=-1
  Gain1 : Gain  Gain=-1
  Gain2 : Gain  Gain=-1
  Saturation : Saturate  UpperLimit=1  LowerLimit=0
  Selector : Selector  InputPortWidth=3  IndexOptions=Index vector (dialog)  Indices=[1]  OutputSizes=1
  Subtract : Sum  Inputs=+-
  Subtract1 : Sum  Inputs=+-
  Stall Stab : Outport
  Yaw Stab : Outport  Port=2
  Pitch Stab : Outport  Port=3
  Roll Stab : Outport  Port=4
  wires:
  Gain2/1 -> Yaw Stab/1
  Bus Selector2/2 -> Selector/1  "<V_b>"
  Discrete Derivative2/1 -> Gain2/1
  Selector/1 -> Subtract/1
  Sensors/1 -> Bus Selector2/1
  Demux/2 -> Discrete Derivative1/1  "theta"
  Demux/1 -> Discrete Derivative/1  "phi"
  Demux/3 -> Discrete Derivative2/1  "psi"
  Discrete Derivative1/1 -> Gain1/1
  Discrete Derivative/1 -> Gain/1
  Bus Selector2/1 -> Demux/1  "<phi_theta_psi>"
  Gain/1 -> Roll Stab/1
  Gain1/1 -> Pitch Stab/1
  Constant1/1 -> Subtract/2
  Saturation/1 -> Stall Stab/1
  Subtract/1 -> Add/1
  Constant/1 -> Add/2
  Add/1 -> Divide/1
  Constant2/1 -> Divide/2
  Divide/1 -> Subtract1/1
  Constant3/1 -> Subtract1/2
  Subtract1/1 -> Saturation/1

== system UAV/Flight Dynamics/6DOF EOM ==
  Bus Element In : Inport  PortName=Env  Element=g
  Forces : Inport  Port=2
  Moments : Inport  Port=3
  6DOF (Euler Angles) : shared6dof/6DOF (Euler Angles)  units=Metric (MKS)  mtype=Fixed  rep=Euler Angles  xme_0=initConditions.x0  Vm_0=initConditions.v0  eul_0=initConditions.euler0  pm_0=initConditions.w0  mass_0=vehicle.mass  mass_e=0.5  mass_f=2.0  inertia=vehicle.inertia  inertia_e=eye(3)  inertia_f=2*eye(3)  k_quat=1.0  vre_flag=on  abi_flag=on  aMode=0  xme_statename={'Xe', 'Ye', 'Ze'}  Vm_statename={'Ubody', 'Vbody', 'Wbody'}  eul_statename={'phi', 'theta', 'psi'}  quat_statename={'qr', 'qi', 'qj','qk'}  pm_statename={'p', 'q', 'r'}  mass_statename=''
      settings: SourceProductBaseCode=AE
  Gain : Gain  Gain=vehicle.mass
  Product : Product  Multiplication=Matrix(*)
  Sum2 : Sum  Inputs=++|  SaturateOnIntegerOverflow=on  InputSameDT=on  OutDataTypeStr=Inherit: Same as first input
  Terminator1 : Terminator
  Terminator2 : Terminator
  Bus Element Out : Outport  PortName=States  Element=euler_angles
  Bus Element Out1 : Outport  PortName=States  Element=omega
  Bus Element Out2 : Outport  PortName=States  Element=omega_dot
  Bus Element Out15 : Outport  PortName=States  Element=X_e
  Bus Element Out16 : Outport  PortName=States  Element=V_b
  Bus Element Out17 : Outport  PortName=States  Element=A_be
  wires:
  6DOF (Euler Angles)/4 -> Product/1
  6DOF (Euler Angles)/1 -> Terminator2/1
  Bus Element In/1 -> Gain/1
  6DOF (Euler Angles)/9 -> Bus Element Out17/1
  6DOF (Euler Angles)/7 -> Bus Element Out2/1
  6DOF (Euler Angles)/6 -> Bus Element Out1/1
  6DOF (Euler Angles)/5 -> Bus Element Out16/1
  6DOF (Euler Angles)/3 -> Bus Element Out/1
  6DOF (Euler Angles)/2 -> Bus Element Out15/1
  Gain/1 -> Product/2
  Moments/1 -> 6DOF (Euler Angles)/2
  Forces/1 -> Sum2/2
  Sum2/1 -> 6DOF (Euler Angles)/1
  Product/1 -> Sum2/1
  6DOF (Euler Angles)/8 -> Terminator1/1

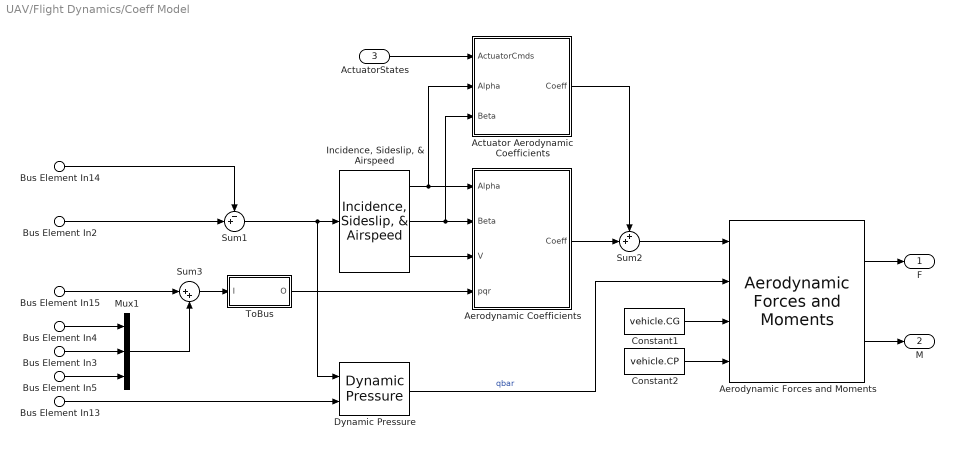
== system UAV/Flight Dynamics/Coeff Model ==
  Bus Element In13 : Inport  PortName=Env  Element=AirDensity
  Bus Element In14 : Inport  PortName=Env  Element=WindVelocity
  Bus Element In15 : Inport  PortName=Env  Element=WindAngularRates
  Bus Element In3 : Inport  Port=2  PortName=States  Element=q
  Bus Element In4 : Inport  Port=2  PortName=States  Element=p
  Bus Element In5 : Inport  Port=2  PortName=States  Element=r
  Bus Element In2 : Inport  Port=2  PortName=States  Element=V_b
  ActuatorStates : Inport  Port=3  OutDataTypeStr=Bus: ActuatorStates
  Actuator Aerodynamic Coefficients : Subsystem
  Aerodynamic Coefficients : Subsystem
  Aerodynamic Forces and Moments : aerolibadyn/Aerodynamic Forces and Moments   inputAxes=Body  outputForceAxes=Body  outputMomentAxes=Body  S=vehicle.wingarea  b=vehicle.wingspan  cbar=vehicle.aclength
      settings: SourceProductName=Aerospace Blockset
  Constant1 : Constant  Value=vehicle.CG
  Constant2 : Constant  Value=vehicle.CP
  Dynamic Pressure : aerolibasang/Dynamic Pressure
  "Incidence, Sideslip, & Airspeed" : aerolibasang/Incidence, Sideslip, & Airspeed
      settings: SourceProductName=Aerospace Blockset
  Mux1 : Mux  Inputs=3
  Sum1 : Sum  Inputs=-+|  SaturateOnIntegerOverflow=on  InputSameDT=on  OutDataTypeStr=Inherit: Same as first input
  Sum2 : Sum  Inputs=++|
  Sum3 : Sum  Inputs=|++  SaturateOnIntegerOverflow=on  InputSameDT=on  OutDataTypeStr=Inherit: Same as first input
  ToBus : Subsystem
  F : Outport  Unit=N
  M : Outport  Port=2  Unit=N*m
  wires:
  ActuatorStates/1 -> Actuator Aerodynamic Coefficients/1(ActuatorCmds)
  Bus Element In14/1 -> Sum1/1
  Bus Element In2/1 -> Sum1/2
  Mux1/1 -> Sum3/2
  Bus Element In15/1 -> Sum3/1
  Bus Element In5/1 -> Mux1/3
  Bus Element In3/1 -> Mux1/2
  Bus Element In4/1 -> Mux1/1
  Actuator Aerodynamic Coefficients/1(Coeff) -> Sum2/1
  Aerodynamic Coefficients/1(Coeff) -> Sum2/2
  ToBus/1(O) -> Aerodynamic Coefficients/4(pqr)
  Sum1/1 -> Dynamic Pressure/1, "Incidence, Sideslip, & Airspeed"/1
  Dynamic Pressure/1 -> Aerodynamic Forces and Moments/2  "qbar"
  Sum3/1 -> ToBus/1(I)
  Bus Element In13/1 -> Dynamic Pressure/2
  "Incidence, Sideslip, & Airspeed"/3 -> Aerodynamic Coefficients/3(V)
  "Incidence, Sideslip, & Airspeed"/2 -> Aerodynamic Coefficients/2(Beta), Actuator Aerodynamic Coefficients/3(Beta)
  Aerodynamic Forces and Moments/2 -> M/1
  Aerodynamic Forces and Moments/1 -> F/1
  Constant2/1 -> Aerodynamic Forces and Moments/4
  Constant1/1 -> Aerodynamic Forces and Moments/3
  Sum2/1 -> Aerodynamic Forces and Moments/1
  "Incidence, Sideslip, & Airspeed"/1 -> Actuator Aerodynamic Coefficients/2(Alpha), Aerodynamic Coefficients/1(Alpha)

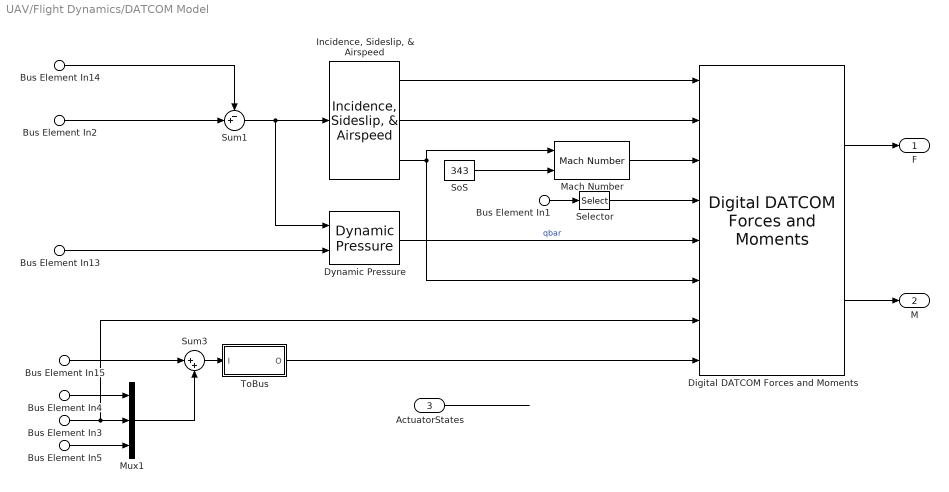
== system UAV/Flight Dynamics/DATCOM Model ==
  Bus Element In13 : Inport  PortName=Env  Element=AirDensity
  Bus Element In14 : Inport  PortName=Env  Element=WindVelocity
  Bus Element In15 : Inport  PortName=Env  Element=WindAngularRates
  Bus Element In3 : Inport  Port=2  PortName=States  Element=q
  Bus Element In4 : Inport  Port=2  PortName=States  Element=p
  Bus Element In5 : Inport  Port=2  PortName=States  Element=r
  Bus Element In2 : Inport  Port=2  PortName=States  Element=V_b
  Bus Element In1 : Inport  Port=2  PortName=States  Element=X_e
  ActuatorStates : Inport  Port=3  OutDataTypeStr=Bus: ActuatorStates
  Digital DATCOM Forces and Moments : aerolibadyn/Digital DATCOM Forces and Moments  units=Metric (MKS)  dcase=datcom{3}  fmode=Wind  buildno=0  imethod=Linear  emethod=None - clip  rmethod=Clip to Range  action=Warning
      settings: SourceProductName=Aerospace Blockset  SourceProductBaseCode=AE
  Dynamic Pressure : aerolibasang/Dynamic Pressure
  "Incidence, Sideslip, & Airspeed" : aerolibasang/Incidence, Sideslip, & Airspeed
      settings: SourceProductName=Aerospace Blockset
  Mach Number : aerolibasang/Mach Number
      settings: SourceProductName=Aerospace Blockset  SourceProductBaseCode=AE
  Mux1 : Mux  Inputs=3
  Selector : Selector  InputPortWidth=3  IndexOptions=Index vector (dialog)  Indices=[3]  OutputSizes=1
  SoS : Constant  Value=343
  Sum1 : Sum  Inputs=-+|  SaturateOnIntegerOverflow=on  InputSameDT=on  OutDataTypeStr=Inherit: Same as first input
  Sum3 : Sum  Inputs=|++  SaturateOnIntegerOverflow=on  InputSameDT=on  OutDataTypeStr=Inherit: Same as first input
  ToBus : Subsystem
  F : Outport  Unit=N
  M : Outport  Port=2  Unit=N*m
  wires:
  ActuatorStates/1 -> ?
  Bus Element In14/1 -> Sum1/1
  Bus Element In2/1 -> Sum1/2
  Mux1/1 -> Sum3/2
  Bus Element In15/1 -> Sum3/1
  Bus Element In5/1 -> Mux1/3
  Bus Element In3/1 -> Digital DATCOM Forces and Moments/7, Mux1/2
  Bus Element In4/1 -> Mux1/1
  ToBus/1(O) -> Digital DATCOM Forces and Moments/8
  Sum1/1 -> Dynamic Pressure/1, "Incidence, Sideslip, & Airspeed"/1
  Sum3/1 -> ToBus/1(I)
  Bus Element In13/1 -> Dynamic Pressure/2
  "Incidence, Sideslip, & Airspeed"/3 -> Mach Number/1, Digital DATCOM Forces and Moments/6
  "Incidence, Sideslip, & Airspeed"/2 -> Digital DATCOM Forces and Moments/2
  Digital DATCOM Forces and Moments/2 -> M/1
  Digital DATCOM Forces and Moments/1 -> F/1
  "Incidence, Sideslip, & Airspeed"/1 -> Digital DATCOM Forces and Moments/1
  Dynamic Pressure/1 -> Digital DATCOM Forces and Moments/5  "qbar"
  Bus Element In1/1 -> Selector/1
  Selector/1 -> Digital DATCOM Forces and Moments/4
  Mach Number/1 -> Digital DATCOM Forces and Moments/3
  SoS/1 -> Mach Number/2

== system UAV/Flight Dynamics/Propulsion ==
  cmd : Inport
  Mux : Mux  Inputs=[1 2]
  Product : Product
  ThrustX : Lookup_n-D  NumberOfTableDimensions=1  LookupTableObject=''  BreakpointsForDimension1=(1/6)*(3+([-3:3]))  IndexSearchMethod=Linear search  BeginIndexSearchUsingPreviousIndexResult=on  Table=vehicle.thrust*(1+tanh([-3:3]))  ExtrapMethod=Clip  InputSameDT=on
  ThrustYZ : Constant  Value=[0 0]'  SampleTime=-1
  Thrust_M1 : Constant  Value=[0 0 0]'  SampleTime=-1
  Vector Concatenate : Concatenate
  F : Outport  Unit=N
  M : Outport  Port=2  Unit=N*m
  wires:
  Thrust_M1/1 -> Product/2
  ThrustX/1 -> Mux/1, Vector Concatenate/2
  ThrustYZ/1 -> Vector Concatenate/1, Mux/2
  Mux/1 -> F/1
  cmd/1 -> ThrustX/1
  Product/1 -> M/1
  Vector Concatenate/1 -> Product/1
